simulink model "TST_StSys_AddCor"  (R2016b)
settings: Solver=FixedStepDiscrete  StartTime=0.0  StopTime=simTime  FixedStep=sampleTime  RelTol=1e-3
values from neighbouring files (symbols this model uses):
  testCase = 1    [initTST_StSys_AddCor_001.m]
libraries: simulink x3, UnitTest_Lib x1
settings Model: Creator=zhengjinyan  LastModifiedBy=zhengjinyan
settings DebuggingCC: SignalRangeChecking=error

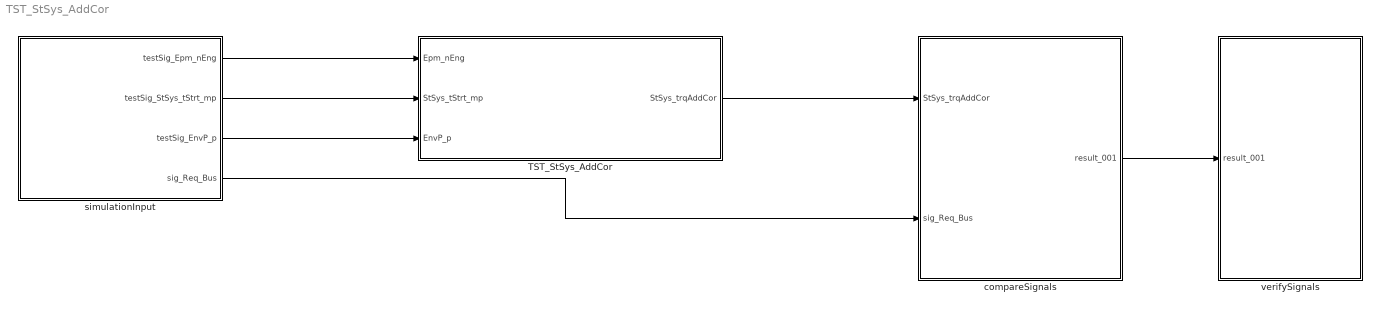
== system TST_StSys_AddCor ==
  TST_StSys_AddCor : Subsystem
  compareSignals : Subsystem
  simulationInput : Subsystem
  verifySignals : Subsystem
  wires:
  simulationInput/1(testSig_Epm_nEng) -> TST_StSys_AddCor/1(Epm_nEng)
  simulationInput/2(testSig_StSys_tStrt_mp) -> TST_StSys_AddCor/2(StSys_tStrt_mp)
  simulationInput/3(testSig_EnvP_p) -> TST_StSys_AddCor/3(EnvP_p)
  TST_StSys_AddCor/1(StSys_trqAddCor) -> compareSignals/1(StSys_trqAddCor)
  simulationInput/4(sig_Req_Bus) -> compareSignals/2(sig_Req_Bus)
  compareSignals/1(result_001) -> verifySignals/1(result_001)

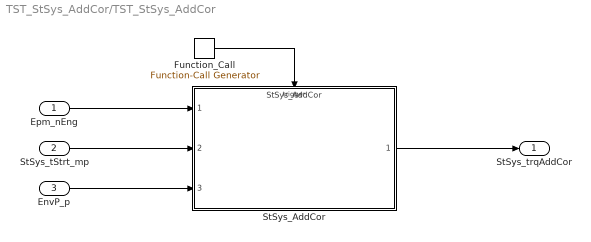
== system TST_StSys_AddCor/TST_StSys_AddCor ==
  Epm_nEng : Inport
  StSys_tStrt_mp : Inport  Port=2
  EnvP_p : Inport  Port=3
  Function_Call : simulink/Ports & Subsystems/Function-Call Generator  sample_time=sampleTime  numberOfIterations=1
  StSys_AddCor : ModelReference  ModelNameDialog=StSys_AddCor  SimulationMode=Normal  ModelReferenceVersion=1.9  TriggerPortName=function  TriggerPortTriggerType=function-call  TriggerPortStatesWhenEnabling=held
  StSys_trqAddCor : Outport
  wires:
  Function_Call/1 -> StSys_AddCor/Trigger
  Epm_nEng/1 -> StSys_AddCor/1
  StSys_tStrt_mp/1 -> StSys_AddCor/2
  EnvP_p/1 -> StSys_AddCor/3
  StSys_AddCor/1 -> StSys_trqAddCor/1

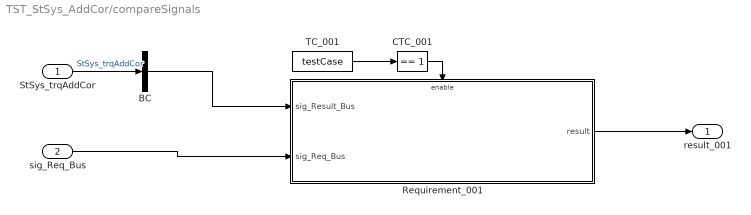
== system TST_StSys_AddCor/compareSignals ==
  StSys_trqAddCor : Inport
  sig_Req_Bus : Inport  Port=2
  BC : BusCreator  Inputs=1
  CTC_001 : simulink/Logic and Bit Operations/Compare To Constant  relop===  const=1  OutDataTypeStr=boolean
  Requirement_001 : Subsystem
  TC_001 : Constant  Value=testCase
  result_001 : Outport
  wires:
  StSys_trqAddCor/1 -> BC/1  "StSys_trqAddCor"
  TC_001/1 -> CTC_001/1
  CTC_001/1 -> Requirement_001/Enable
  sig_Req_Bus/1 -> Requirement_001/2(sig_Req_Bus)
  BC/1 -> Requirement_001/1(sig_Result_Bus)
  Requirement_001/1(result) -> result_001/1

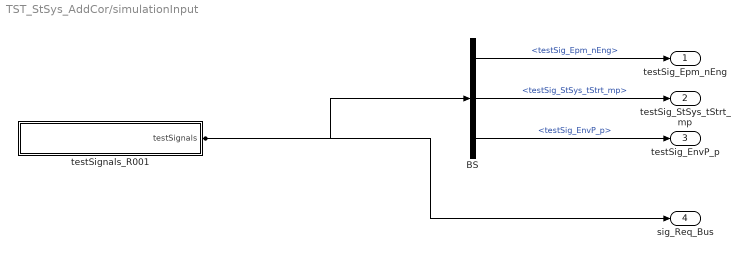
== system TST_StSys_AddCor/simulationInput ==
  BS : BusSelector  OutputSignals=testSig_Epm_nEng,testSig_StSys_tStrt_mp,testSig_EnvP_p
  testSignals_R001 : Subsystem
  testSig_Epm_nEng : Outport
  testSig_StSys_tStrt_mp : Outport  Port=2
  testSig_EnvP_p : Outport  Port=3
  sig_Req_Bus : Outport  Port=4
  wires:
  BS/1 -> testSig_Epm_nEng/1  "<testSig_Epm_nEng>"
  BS/2 -> testSig_StSys_tStrt_mp/1  "<testSig_StSys_tStrt_mp>"
  BS/3 -> testSig_EnvP_p/1  "<testSig_EnvP_p>"
  testSignals_R001/1(testSignals) -> BS/1, sig_Req_Bus/1

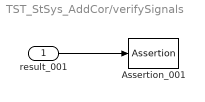
== system TST_StSys_AddCor/verifySignals ==
  result_001 : Inport
  Assertion_001 : Assertion  Enabled=off
  wires:
  result_001/1 -> Assertion_001/1

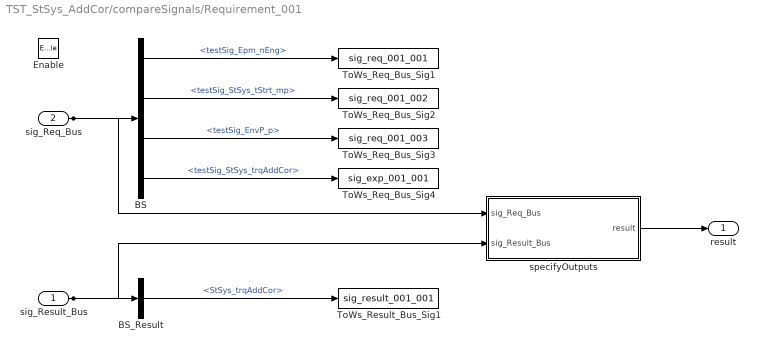
== system TST_StSys_AddCor/compareSignals/Requirement_001 ==
  sig_Result_Bus : Inport
  sig_Req_Bus : Inport  Port=2
  Enable : EnablePort
  BS : BusSelector  OutputSignals=testSig_Epm_nEng,testSig_StSys_tStrt_mp,testSig_EnvP_p,testSig_StSys_trqAddCor
  BS_Result : BusSelector  OutputSignals=StSys_trqAddCor
  ToWs_Req_Bus_Sig1 : ToWorkspace  VariableName=sig_req_001_001  SaveFormat=Structure With Time
  ToWs_Req_Bus_Sig2 : ToWorkspace  VariableName=sig_req_001_002  SaveFormat=Structure With Time
  ToWs_Req_Bus_Sig3 : ToWorkspace  VariableName=sig_req_001_003  SaveFormat=Structure With Time
  ToWs_Req_Bus_Sig4 : ToWorkspace  VariableName=sig_exp_001_001  SaveFormat=Structure With Time
  ToWs_Result_Bus_Sig1 : ToWorkspace  VariableName=sig_result_001_001  SaveFormat=Structure With Time
  specifyOutputs : Subsystem
  result : Outport
  wires:
  sig_Req_Bus/1 -> BS/1, specifyOutputs/1(sig_Req_Bus)
  BS/1 -> ToWs_Req_Bus_Sig1/1  "<testSig_Epm_nEng>"
  BS/2 -> ToWs_Req_Bus_Sig2/1  "<testSig_StSys_tStrt_mp>"
  BS/3 -> ToWs_Req_Bus_Sig3/1  "<testSig_EnvP_p>"
  BS/4 -> ToWs_Req_Bus_Sig4/1  "<testSig_StSys_trqAddCor>"
  sig_Result_Bus/1 -> BS_Result/1, specifyOutputs/2(sig_Result_Bus)
  BS_Result/1 -> ToWs_Result_Bus_Sig1/1  "<StSys_trqAddCor>"
  specifyOutputs/1(result) -> result/1

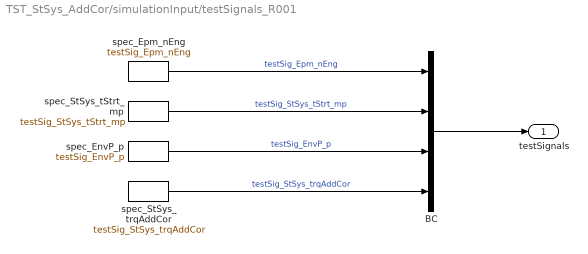
== system TST_StSys_AddCor/simulationInput/testSignals_R001 ==
  BC : BusCreator  Inputs=4
  spec_EnvP_p : FromWorkspace  VariableName=testSig_EnvP_p  Interpolate=off  OutputAfterFinalValue=Holding final value
  spec_Epm_nEng : FromWorkspace  VariableName=testSig_Epm_nEng  Interpolate=off  OutputAfterFinalValue=Holding final value
  spec_StSys_tStrt_mp : FromWorkspace  VariableName=testSig_StSys_tStrt_mp  Interpolate=off  OutputAfterFinalValue=Holding final value
  spec_StSys_trqAddCor : FromWorkspace  VariableName=testSig_StSys_trqAddCor  Interpolate=off  OutputAfterFinalValue=Holding final value
  testSignals : Outport
  wires:
  BC/1 -> testSignals/1
  spec_Epm_nEng/1 -> BC/1  "testSig_Epm_nEng"
  spec_StSys_tStrt_mp/1 -> BC/2  "testSig_StSys_tStrt_mp"
  spec_EnvP_p/1 -> BC/3  "testSig_EnvP_p"
  spec_StSys_trqAddCor/1 -> BC/4  "testSig_StSys_trqAddCor"

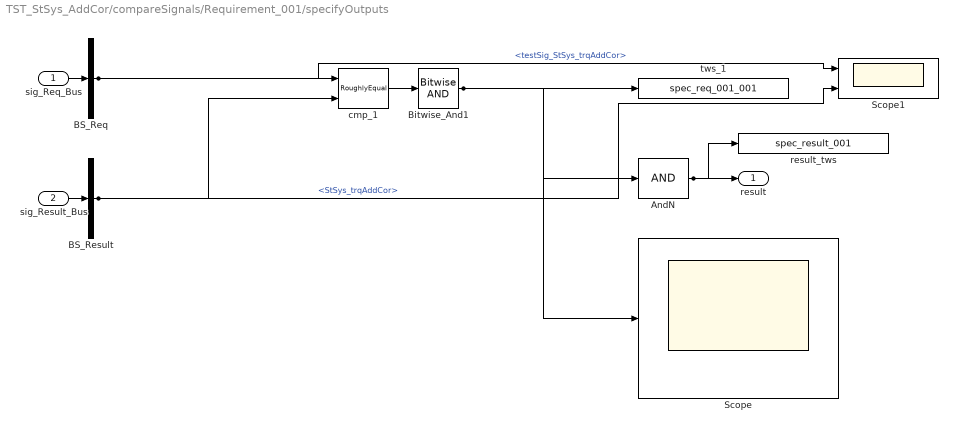
== system TST_StSys_AddCor/compareSignals/Requirement_001/specifyOutputs ==
  sig_Req_Bus : Inport
  sig_Result_Bus : Inport  Port=2
  AndN : Logic  Inputs=1
  BS_Req : BusSelector  OutputSignals=testSig_StSys_trqAddCor
  BS_Result : BusSelector  OutputSignals=StSys_trqAddCor
  Bitwise_And1 : simulink/Logic and Bit Operations/Bitwise Operator  logicop=AND  UseBitMask=off  BitMask=bin2dec('11011001')  BitMaskRealWorld=Stored Integer
  Scope : Scope
  Scope1 : Scope  NumInputPorts=2
  cmp_1 : UnitTest_Lib/RoughlyEqual  slope=0.1
  result_tws : ToWorkspace  VariableName=spec_result_001
  tws_1 : ToWorkspace  VariableName=spec_req_001_001
  result : Outport
  wires:
  sig_Req_Bus/1 -> BS_Req/1
  sig_Result_Bus/1 -> BS_Result/1
  AndN/1 -> result/1, result_tws/1
  BS_Req/1 -> cmp_1/1, Scope1/1  "<testSig_StSys_trqAddCor>"
  BS_Result/1 -> cmp_1/2, Scope1/2  "<StSys_trqAddCor>"
  cmp_1/1 -> Bitwise_And1/1
  Bitwise_And1/1 -> tws_1/1, AndN/1, Scope/1
